simulink model "audio_gen_simulink"  (R2024b)
settings: Solver=VariableStepAuto  StartTime=0.0  StopTime=1  RelTol=1e-3
values from neighbouring files (symbols this model uses):
  f_au = 48e3    (= 48000)    [duc_data_gen.m]
  fs = 120e6    (= 120000000)    [duc_data_analyse.m]    (also in duc_data_gen.m)
  length_score_music = length(vec_score_music)    [audio_gen.m]
  sample_times_one_note = fix(time_one_note*f_au)    [audio_gen.m]
  up_L = fs/f_au    (= 2500)    [duc_data_gen.m]
libraries: hdlsllib x7, simulink x3, dsphdlsigops2 x2, dspvision x1
settings Model: Creator=31651  LastModifiedBy=31651

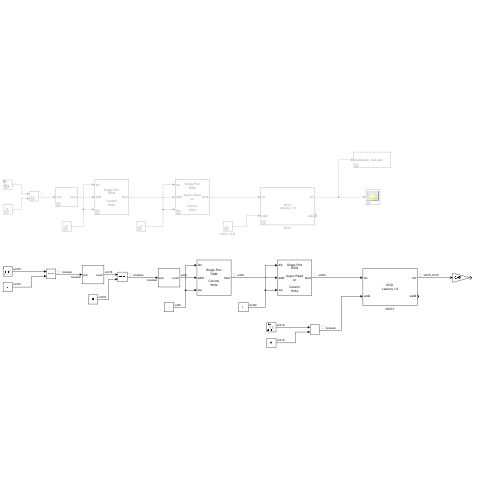
[thumbnail: Simulink's stored preview of the top-level diagram]
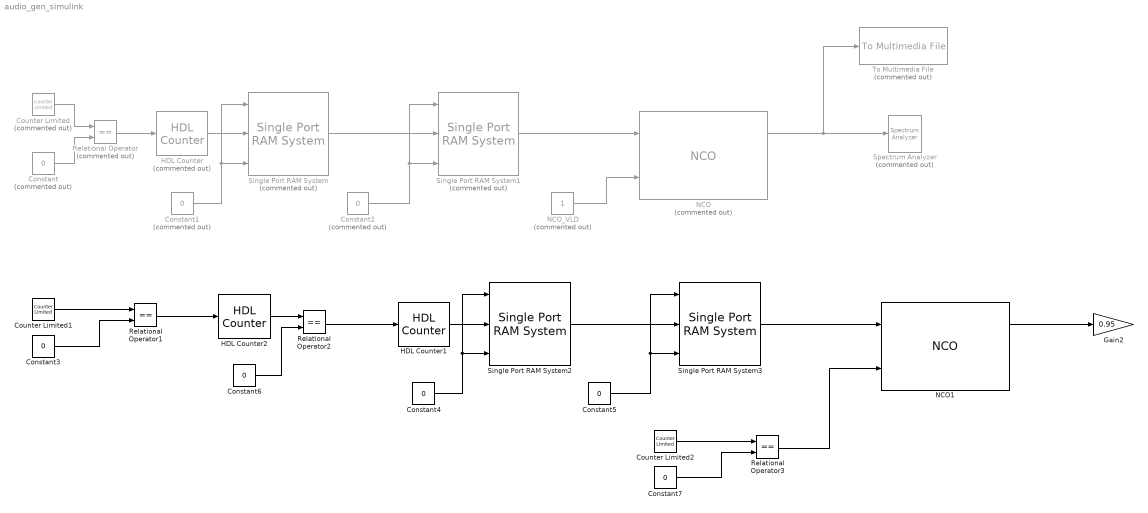
== system audio_gen_simulink ==
  Constant : Constant  Commented=on  Value=0  OutDataTypeStr=uint16  SampleTime=1/f_au
  Constant1 : Constant  Commented=on  Value=0  OutDataTypeStr=uint8  SampleTime=1/f_au
  Constant2 : Constant  Commented=on  Value=0  OutDataTypeStr=uint32  SampleTime=1/f_au
  Constant3 : Constant  Value=0  OutDataTypeStr=uint16  SampleTime=1/fs
  Constant4 : Constant  Value=0  OutDataTypeStr=uint8  SampleTime=1/fs
  Constant5 : Constant  Value=0  OutDataTypeStr=uint32  SampleTime=1/fs
  Constant6 : Constant  Value=0  OutDataTypeStr=uint16  SampleTime=1/fs
  Constant7 : Constant  Value=0  OutDataTypeStr=uint16  SampleTime=1/fs
  Counter Limited : simulink/Sources/Counter Limited  Commented=on  uplimit=sample_times_one_note-1  tsamp=1/f_au
  Counter Limited1 : simulink/Sources/Counter Limited  uplimit=up_L-1  tsamp=1/fs
  Counter Limited2 : simulink/Sources/Counter Limited  uplimit=up_L-1  tsamp=1/fs
  Gain2 : Gain  Gain=0.95  OutDataTypeStr=fixdt(1,16,15)
  HDL Counter : hdlsllib/Sources/HDL Counter  Commented=on  CountType=Count limited  CountInit=0  CountStep=1  CountMax=length_score_music-1  CountFromType=Initial value  CountFrom=0  CountResetPort=off  CountLoadPort=off  CountEnbPort=on  CountDirPort=off  CountHitOutputPort=off  CountDataType=Unsigned  CountWordLen=8  CountFracLen=0  CountSampTime=1/f_au
  HDL Counter1 : hdlsllib/Sources/HDL Counter  CountType=Count limited  CountInit=0  CountStep=1  CountMax=length_score_music-1  CountFromType=Initial value  CountFrom=0  CountResetPort=off  CountLoadPort=off  CountEnbPort=on  CountDirPort=off  CountHitOutputPort=off  CountDataType=Unsigned  CountWordLen=8  CountFracLen=0  CountSampTime=1/f_au
  HDL Counter2 : hdlsllib/Sources/HDL Counter  CountType=Count limited  CountInit=0  CountStep=1  CountMax=sample_times_one_note-1  CountFromType=Initial value  CountFrom=0  CountResetPort=off  CountLoadPort=off  CountEnbPort=on  CountDirPort=off  CountHitOutputPort=off  CountDataType=Unsigned  CountWordLen=16  CountFracLen=0  CountSampTime=1/f_au
  NCO : dsphdlsigops2/NCO  Commented=on  PhaseIncrementSource=Input port  PhaseIncrement=100  PhaseOffsetSource=Property  PhaseOffset=0  DitherSource=Property  NumDitherBits=ditherBits  SamplesPerFrame=1  LUTCompress=on  ResetAction=off  Waveform=Sine  PhasePort=off  SimulateUsing=Code generation  AccumulatorWL=Nnco  PhaseQuantization=on  NumQuantizerAccumulatorBits=Q  OutputDataType=Binary point scaling  OutputWL=16  OutputFL=15
      settings: LibrarySourceBlock=dsphdlsrcs2/NCO
  NCO1 : dsphdlsigops2/NCO  PhaseIncrementSource=Input port  PhaseIncrement=100  PhaseOffsetSource=Property  PhaseOffset=0  DitherSource=Property  NumDitherBits=ditherBits  SamplesPerFrame=1  LUTCompress=on  ResetAction=off  Waveform=Sine  PhasePort=off  SimulateUsing=Code generation  AccumulatorWL=Nnco  PhaseQuantization=on  NumQuantizerAccumulatorBits=Q  OutputDataType=Binary point scaling  OutputWL=16  OutputFL=15
      settings: LibrarySourceBlock=dsphdlsrcs2/NCO
  NCO_VLD : Constant  Commented=on  OutDataTypeStr=boolean  SampleTime=1/f_au
  Relational Operator : RelationalOperator  Commented=on  Operator===  OutDataTypeStr=boolean  RndMeth=Simplest  InputSameDT=off
  Relational Operator1 : RelationalOperator  Operator===  OutDataTypeStr=boolean  RndMeth=Simplest  InputSameDT=off
  Relational Operator2 : RelationalOperator  Operator===  OutDataTypeStr=boolean  RndMeth=Simplest  InputSameDT=off
  Relational Operator3 : RelationalOperator  Operator===  OutDataTypeStr=boolean  RndMeth=Simplest  InputSameDT=off
  Single Port RAM System : hdlsllib/HDL RAMs/Single Port RAM System  Commented=on  RAMType=Single port  AsyncRead=off  WriteOutputValue=New data  RAMInitialValue=vec_score_music  allowBusInputs=off  WritesHaveOutput=on  NumReads=0  NumWrites=1  SimulateUsing=Code generation  ModelRAMDelay=on
  Single Port RAM System1 : hdlsllib/HDL RAMs/Single Port RAM System  Commented=on  RAMType=Single port  AsyncRead=on  WriteOutputValue=New data  RAMInitialValue=vec_freq_music_phinc  allowBusInputs=off  WritesHaveOutput=on  NumReads=0  NumWrites=1  SimulateUsing=Code generation  ModelRAMDelay=on
  Single Port RAM System2 : hdlsllib/HDL RAMs/Single Port RAM System  RAMType=Single port  AsyncRead=off  WriteOutputValue=New data  RAMInitialValue=vec_score_music  allowBusInputs=off  WritesHaveOutput=on  NumReads=0  NumWrites=1  SimulateUsing=Code generation  ModelRAMDelay=on
  Single Port RAM System3 : hdlsllib/HDL RAMs/Single Port RAM System  RAMType=Single port  AsyncRead=on  WriteOutputValue=New data  RAMInitialValue=vec_freq_music_phinc  allowBusInputs=off  WritesHaveOutput=on  NumReads=0  NumWrites=1  SimulateUsing=Code generation  ModelRAMDelay=on
  Spectrum Analyzer : SpectrumAnalyzer  Commented=on  WindowPosition=[305.000000,113.000000,1041.000000,586.000000,]  ScopeFrameLocation=window  WindowInvariantSamplesPerUpdate=on  FrequencySpan=Start and stop frequencies  Span=48000  StartFrequency=-24000  StopFrequency=24000  YLimits=[-90.27739342,38.95560182]  ExpandToolstrip=on  SelectedToolstripTab=spectrumAnalyzerToolstrip.estimationTab
  To Multimedia File : dspvision/To Multimedia File  Commented=on  outputFilename=audio_test.wav  streamSelection=Audio only  videoCompressor=None (uncompressed)  audioCompressor=None (uncompressed)  imagePorts=One multidimensional signal  fileType=WAV  audioDatatype=16-bit integer  fourcc=RGB  audioBitRate=128  audioQuality=75  videoQuality=75  mj2000CompFactor=10
      settings: LibrarySourceBlock=audiosinks/To Multimedia File
  wires:
  Counter Limited/1 -> Relational Operator/1
  Constant/1 -> Relational Operator/2
  Relational Operator/1 -> HDL Counter/1
  HDL Counter/1 -> Single Port RAM System/2
  Constant1/1 -> Single Port RAM System/1, Single Port RAM System/3
  Single Port RAM System/1 -> Single Port RAM System1/2
  Constant2/1 -> Single Port RAM System1/3, Single Port RAM System1/1
  Single Port RAM System1/1 -> NCO/1
  NCO_VLD/1 -> NCO/2
  NCO/1 -> To Multimedia File/1, Spectrum Analyzer/1
  HDL Counter2/1 -> Relational Operator2/1
  Counter Limited1/1 -> Relational Operator1/1
  Constant3/1 -> Relational Operator1/2
  Relational Operator2/1 -> HDL Counter1/1
  Constant6/1 -> Relational Operator2/2
  NCO1/1 -> Gain2/1
  Constant5/1 -> Single Port RAM System3/3, Single Port RAM System3/1
  Single Port RAM System2/1 -> Single Port RAM System3/2
  Relational Operator1/1 -> HDL Counter2/1
  Constant4/1 -> Single Port RAM System2/1, Single Port RAM System2/3
  Single Port RAM System3/1 -> NCO1/1
  HDL Counter1/1 -> Single Port RAM System2/2
  Relational Operator3/1 -> NCO1/2
  Counter Limited2/1 -> Relational Operator3/1
  Constant7/1 -> Relational Operator3/2
